simulink library "simpleDragTurbine_ul"  (R2018b)
settings: Solver=VariableStepAuto  StartTime=0.0  StopTime=10.0  RelTol=1e-3
values from neighbouring files (symbols this model uses):
  rho_fluid = 1    [simpleDragTurbine_ts.m]
undefined symbols (not defined in the file or in its folder): attchPts, Cds, Cps, dias, nTurbines, turbine
libraries: vrlib x1, eulAng2RotMat_ul x1, vectorDirection x1
settings Model: Creator=Ayaz  LastModifiedBy=Ayaz

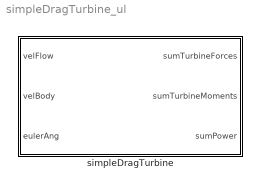
== system simpleDragTurbine_ul ==
  simpleDragTurbine : Subsystem  TreatAsAtomicUnit=on  mask{rho_fluid=rho_fluid, turb_struct=turbine}
      mask prompts: rho_fluid "Fluid density"; turb_struct "Turbines structure"
      mask init:
      | simpleDragTurbine_init

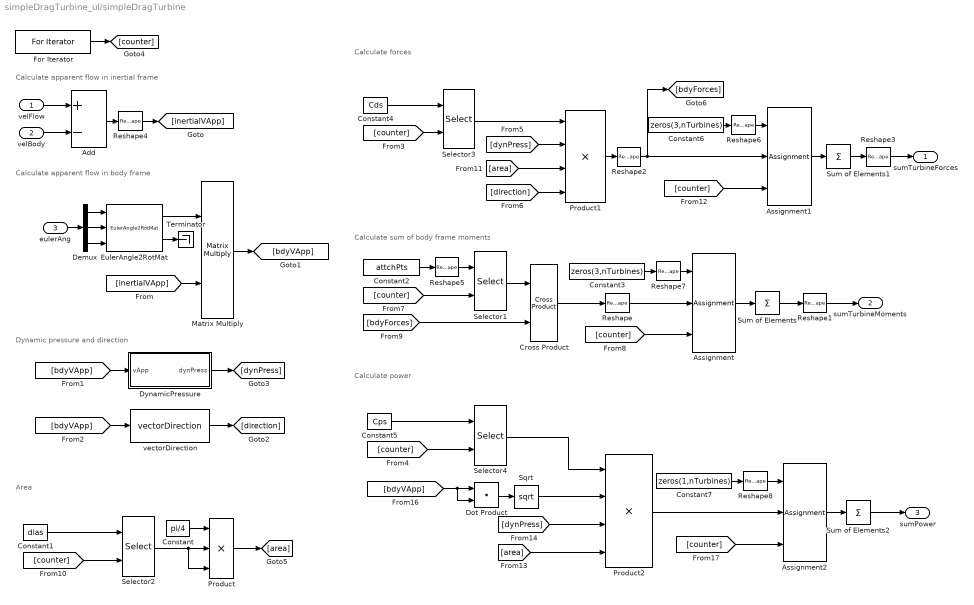
== system simpleDragTurbine_ul/simpleDragTurbine ==
  note: Calculate apparent flow in inertial frame
  note: Area
  note: Calculate apparent flow in body frame
  note: Calculate forces
  note: Calculate power
  note: Dynamic pressure and direction
  note: Calculate sum of body frame moments
  velFlow : Inport
  velBody : Inport  Port=2
  eulerAng : Inport  Port=3
  Add : Sum  Inputs=+-
  Assignment : Assignment  NumberOfDimensions=2  DiagnosticForDimensions=Warning  IndexOptions=Assign all,Index vector (port)  Indices=1,1  OutputSizes=1,1
  Assignment1 : Assignment  NumberOfDimensions=2  DiagnosticForDimensions=Warning  IndexOptions=Assign all,Index vector (port)  Indices=1,1  OutputSizes=1,1
  Assignment2 : Assignment  DiagnosticForDimensions=Warning  IndexOptions=Index vector (port)  Indices=1  OutputSizes=1
  Constant : Constant  Value=pi/4
  Constant1 : Constant  Value=dias
  Constant2 : Constant  Value=attchPts
  Constant3 : Constant  Value=zeros(3,nTurbines)
  Constant4 : Constant  Value=Cds
  Constant5 : Constant  Value=Cps
  Constant6 : Constant  Value=zeros(3,nTurbines)
  Constant7 : Constant  Value=zeros(1,nTurbines)
  Cross Product : vrlib/Utilities/Cross Product
      settings: SourceProductBaseCode=VR
  Demux : Demux  Outputs=3
  Dot Product : DotProduct  InputSameDT=on  OutDataTypeStr=Inherit: Inherit via internal rule
  DynamicPressure : Subsystem  mask{rho=rho_fluid}
      mask prompts: rho "Fluid density"
  EulerAngle2RotMat : eulAng2RotMat_ul/EulerAngle2RotMat  SystemSampleTime=-1
  For Iterator : ForIterator  IterationLimit=nTurbines
  Matrix Multiply : Product  Multiplication=Matrix(*)
  Product : Product  Inputs=3
  Product1 : Product  Inputs=4
  Product2 : Product  Inputs=4
  Reshape{,1..4} (5 alike) : Reshape  OutputDimensionality=Column vector (2-D)
  Reshape5 : Reshape  OutputDimensionality=Customize  OutputDimensions=[3,nTurbines]
  Reshape6 : Reshape  OutputDimensionality=Customize  OutputDimensions=[3,nTurbines]
  Reshape7 : Reshape  OutputDimensionality=Customize  OutputDimensions=[3,nTurbines]
  Reshape8 : Reshape  OutputDimensionality=Row vector (2-D)  OutputDimensions=[3,nTurbines]
  Selector1 : Selector  NumberOfDimensions=2  InputPortWidth=3  IndexOptions=Select all,Index vector (port)  Indices=[1 3],1  OutputSizes=1,1
  Selector2 : Selector  NumberOfDimensions=2  InputPortWidth=1  IndexOptions=Select all,Index vector (port)  Indices=[1 3],1  OutputSizes=1,1
  Selector3 : Selector  NumberOfDimensions=2  InputPortWidth=1  IndexOptions=Select all,Index vector (port)  Indices=[1 3],1  OutputSizes=1,1
  Selector4 : Selector  NumberOfDimensions=2  InputPortWidth=1  IndexOptions=Select all,Index vector (port)  Indices=[1 3],1  OutputSizes=1,1
  Sqrt : Sqrt  SaturateOnIntegerOverflow=on
  Sum of Elements : Sum  Inputs=+  CollapseMode=Specified dimension  CollapseDim=2
  Sum of Elements1 : Sum  Inputs=+  CollapseMode=Specified dimension  CollapseDim=2
  Sum of Elements2 : Sum  Inputs=+  CollapseMode=Specified dimension  CollapseDim=2
  Terminator : Terminator
  vectorDirection : vectorDirection/vectorDirection  SystemSampleTime=-1
  sumTurbineForces : Outport
  sumTurbineMoments : Outport  Port=2
  sumPower : Outport  Port=3
  wires:
  velBody/1 -> Add/2
  velFlow/1 -> Add/1
  DynamicPressure/1(dynPress) -> [dynPress]
  vectorDirection/1 -> [direction]
  Matrix Multiply/1 -> [bdyVApp]
  [bdyVApp] -> DynamicPressure/1(vApp)
  EulerAngle2RotMat/2 -> Terminator/1
  eulerAng/1 -> Demux/1
  Demux/3 -> EulerAngle2RotMat/3
  EulerAngle2RotMat/1 -> Matrix Multiply/1
  Demux/2 -> EulerAngle2RotMat/2
  Demux/1 -> EulerAngle2RotMat/1
  [bdyVApp] -> vectorDirection/1
  [inertialVApp] -> Matrix Multiply/2
  For Iterator/1 -> [counter]
  [counter] -> Selector1/2
  Cross Product/1 -> Reshape/1
  [counter] -> Assignment/3
  Reshape1/1 -> sumTurbineMoments/1
  Reshape/1 -> Assignment/2
  Selector1/1 -> Cross Product/1
  Constant2/1 -> Reshape5/1
  Assignment/1 -> Sum of Elements/1
  Sum of Elements/1 -> Reshape1/1
  [bdyForces] -> Cross Product/2
  Selector2/1 -> Product/3, Product/2
  Constant/1 -> Product/1
  Product/1 -> [area]
  [counter] -> Selector4/2
  [counter] -> Selector3/2
  Selector3/1 -> Product1/1
  [dynPress] -> Product1/2
  [area] -> Product1/3
  [direction] -> Product1/4
  [counter] -> Assignment1/3
  Assignment1/1 -> Sum of Elements1/1
  Reshape2/1 -> [bdyForces], Assignment1/2
  Product1/1 -> Reshape2/1
  Constant6/1 -> Reshape6/1
  Sum of Elements1/1 -> Reshape3/1
  Reshape3/1 -> sumTurbineForces/1
  [bdyVApp] -> Dot Product/2, Dot Product/1
  Dot Product/1 -> Sqrt/1
  Selector4/1 -> Product2/1
  [area] -> Product2/4
  [dynPress] -> Product2/3
  Sqrt/1 -> Product2/2
  [counter] -> Assignment2/3
  Assignment2/1 -> Sum of Elements2/1
  Product2/1 -> Assignment2/2
  Sum of Elements2/1 -> sumPower/1
  Add/1 -> Reshape4/1
  Reshape4/1 -> [inertialVApp]
  [counter] -> Selector2/2
  Constant1/1 -> Selector2/1
  Constant4/1 -> Selector3/1
  Reshape5/1 -> Selector1/1
  Reshape6/1 -> Assignment1/1
  Constant3/1 -> Reshape7/1
  Reshape7/1 -> Assignment/1
  Constant7/1 -> Reshape8/1
  Reshape8/1 -> Assignment2/1
  Constant5/1 -> Selector4/1

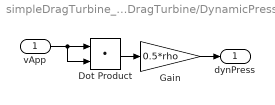
== system simpleDragTurbine_ul/simpleDragTurbine/DynamicPressure ==
  vApp : Inport
  Dot Product : DotProduct  InputSameDT=on  OutDataTypeStr=Inherit: Inherit via internal rule
  Gain : Gain  Gain=0.5*rho
  dynPress : Outport
  wires:
  Gain/1 -> dynPress/1
  vApp/1 -> Dot Product/2, Dot Product/1
  Dot Product/1 -> Gain/1
